simulink model "ntau_"  (R2015a)
settings: Solver=FixedStepDiscrete  StartTime=0.0  StopTime=1.0  FixedStep=1.0  RelTol=1e-3
libraries: taXlibrary x7
settings Model: Creator=emmert  LastModifiedBy=thomas
settings DataIOCC: SignalLoggingSaveFormat=ModelDataLogs
settings OptimizationCC: ExpressionDepthLimit=2147483647
settings DebuggingCC: UnderspecifiedInitializationDetection=Classic  MergeDetectMultiDrivingBlocksExec=none  SolverPrmCheckMsg=warning  FcnCallInpInsideContextMsg=EnableAllAsWarning  StateNameClashWarn=warning
settings GRTTargetCC: CombineOutputUpdateFcns=off  GRTInterface=on

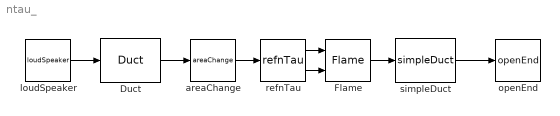
== system ntau_ ==
  Duct : taXlibrary/Duct  element=Duct  order=3  minres=40  l=0.5  sensorPositions=[]
      settings: AttributesFormatString=%<l> m
  Flame : taXlibrary/Flame  element=rankineHugoniot  nRef=1  Mach=0.001056*101325/(287.04*293)*11.3/(101325/(287.04*1930)*0.0081*sqrt(1.4*287.04*1930))  rho=101325/(287.04*1930)  c=sqrt(1.4*287.04*1930)
  areaChange : taXlibrary/areaChange  element=lZeta  zeta=0  lred=0  leff=0  l=1  A=4
      settings: AttributesFormatString=%<A> m^2
  loudSpeaker : taXlibrary/loudSpeaker  element=loudSpeaker  loc=Upstream  Amp=1  A=1.4  Mach=0.1  rho=1.2  c=100
      settings: AttributesFormatString=%<Amp> m/s
  openEnd : taXlibrary/openEnd  element=openEnd  loc=Downstream  A=[]  Mach=[]  rho=[]  c=[]
  refnTau : taXlibrary/refnTau  element=reference  n=1  tau=0.01  active=on  filename=FTF_ntau.m  modelname=0
  simpleDuct : taXlibrary/simpleDuct  element=simpleDuct  l=0.25  damping_model_popup=no damping  gm=1.4  nu=1.568e-5  Pr=5  damping_model_id=1
      settings: AttributesFormatString=%<l> m
  wires:
  loudSpeaker/1 -> Duct/1
  simpleDuct/1 -> openEnd/1
  Duct/1 -> areaChange/1
  areaChange/1 -> refnTau/1
  refnTau/1 -> Flame/1
  refnTau/2 -> Flame/2
  Flame/1 -> simpleDuct/1
